simulink model "model_2"  (R2018b)
settings: Solver=VariableStepAuto  StartTime=0.0  StopTime=10.0  RelTol=1e-3
values from neighbouring files (symbols this model uses):
  A_2 = A'    [zad1.m]
  B_2 = C'    [zad1.m]
settings Model: Creator=mariu  LastModifiedBy=mariu

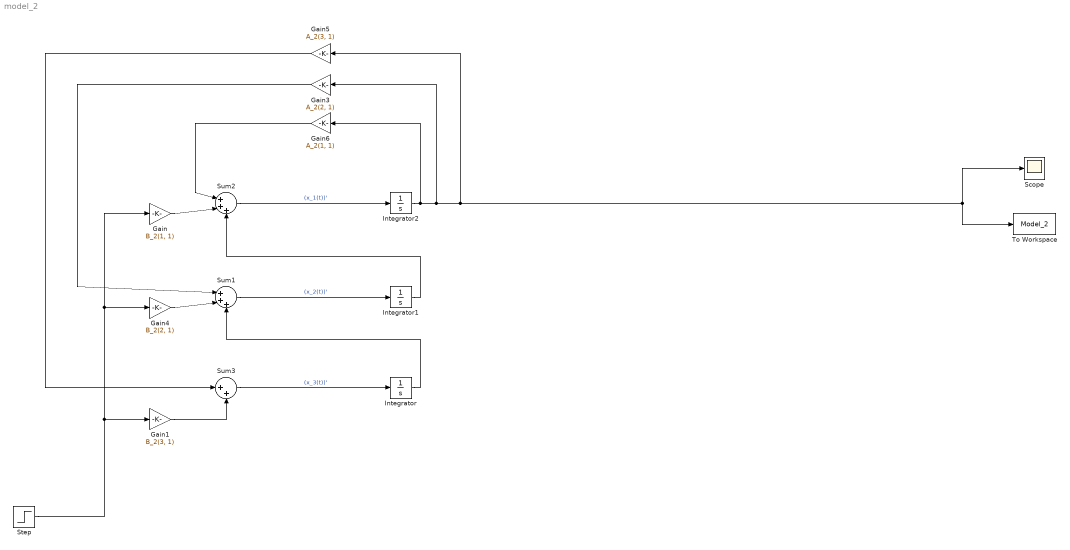
== system model_2 ==
  Gain : Gain  Gain=B_2(1, 1)
  Gain1 : Gain  Gain=B_2(3, 1)
  Gain3 : Gain  Gain=A_2(2, 1)
  Gain4 : Gain  Gain=B_2(2, 1)
  Gain5 : Gain  Gain=A_2(3, 1)
  Gain6 : Gain  Gain=A_2(1, 1)
  Integrator : Integrator
  Integrator1 : Integrator
  Integrator2 : Integrator
  Scope : Scope
  Step : Step  SampleTime=0
  Sum1 : Sum  Inputs=|+++
      settings: AttributesFormatString=%<Inputs>
  Sum2 : Sum  Inputs=|+++
      settings: AttributesFormatString=%<Inputs>
  Sum3 : Sum  Inputs=|++
      settings: AttributesFormatString=%<Inputs>
  To Workspace : ToWorkspace  VariableName=Model_2  SaveFormat=Timeseries  SampleTime=-1
  wires:
  Integrator2/1 -> Gain3/1, Gain5/1, Scope/1, To Workspace/1, Gain6/1
  Sum2/1 -> Integrator2/1  "(x_1(t))'"
  Step/1 -> Gain/1, Gain4/1, Gain1/1
  Gain6/1 -> Sum2/1
  Gain/1 -> Sum2/2
  Integrator1/1 -> Sum2/3
  Sum1/1 -> Integrator1/1  "(x_2(t))'"
  Integrator/1 -> Sum1/3
  Gain3/1 -> Sum1/1
  Gain4/1 -> Sum1/2
  Gain5/1 -> Sum3/1
  Gain1/1 -> Sum3/2
  Sum3/1 -> Integrator/1  "(x_3(t))'"
